simulink model "FSFBlinear"  (R2023a)
settings: Solver=ode45  StartTime=0.0  StopTime=100  RelTol=1e-8  AbsTol=1e-8
values from neighbouring files (symbols this model uses):
  epsc = -epsc    [FEEDBACK_ODE.m]    (also in HW5.m = epsc2)
  etac = etac2    [HW5.m]
  I = diag([1200 2000 2800])    [HW5.m]
  kd = -kd    [HW5.m]
  kp = -kp    [HW5.m]
  X0 = [eps0;w0]    [HW5.m]
settings Model: Creator=Josh2  LastModifiedBy=Josh2
settings ModelReferenceCC: EnableRefExpFcnMdlSchedulingChecks=on

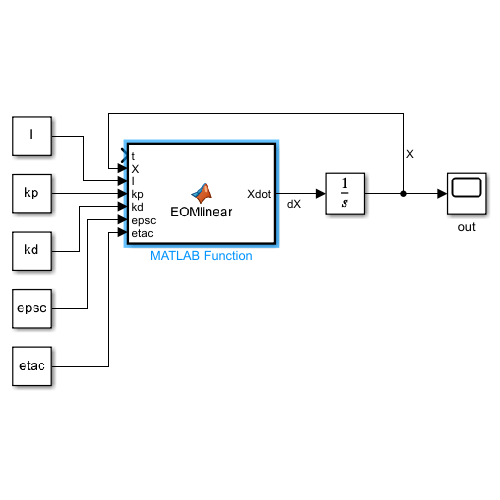
[thumbnail: Simulink's stored preview of the top-level diagram]
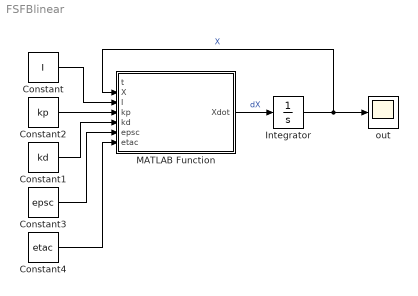
== system FSFBlinear ==
  Constant : Constant  Value=I
  Constant1 : Constant  Value=kd
  Constant2 : Constant  Value=kp
  Constant3 : Constant  Value=epsc
  Constant4 : Constant  Value=etac
  Integrator : Integrator  InitialCondition=X0
  MATLAB Function : MATLAB Function  TreatAsAtomicUnit=on
  out : Scope
  wires:
  MATLAB Function/1(Xdot) -> Integrator/1  "dX"
  Integrator/1 -> out/1, MATLAB Function/2(X)  "X"
  Constant/1 -> MATLAB Function/3(I)
  Constant2/1 -> MATLAB Function/4(kp)
  Constant1/1 -> MATLAB Function/5(kd)
  Constant3/1 -> MATLAB Function/6(epsc)
  Constant4/1 -> MATLAB Function/7(etac)

== matlab function FSFBlinear/MATLAB Function ==
  data: t input; Xdot output; X input; I input; kp input; kd input; epsc input; etac input
function Xdot = EOMlinear(t,X,I,kp,kd,epsc,etac)
% pass through function calls shared ODE (because this is the world we live in)
Xdot = zeros(6,1);
Xdot = EOM_ODElinear(t,X,I,kp,kd,epsc,etac);
end
